simulink model "Kalman_offline_sim"  (R2022b)
settings: Solver=VariableStepAuto  StartTime=0.0  StopTime=sim_time-0.02  RelTol=1e-3
values from neighbouring files (symbols this model uses):
  A_d = (eye(size(A))+Ts*A)    [Kalman_offline.m]    (also in Main_sim.m; Startup_labview.m)
  B_d = Ts*B    [Kalman_offline.m]    (also in Main_sim.m; Startup_labview.m)
  bike_params = LoadBikeParameters(bike)    [Kalman_offline.m]    (also in Main_sim.m; Startup_labview.m)
  C1 = [1 0 0 0 0 0 0 ... (first row only)    [Kalman_offline.m]    (also in Main_sim.m; Startup_labview.m)
  C2 = [(-g+((-h_imu*g)/h)) 0 (-h_imu*(h*v^2-(g*lr*c)))*sin(lambda)/((lr+lf)*h^2)+(v^2)*sin(lambda)/(lr+lf) 0 ... (first row only)    [Kalman_offline.m]    (also in Main_sim.m; Startup_labview.m)
  D1 = [0 0 (-h_imu*lr*v)/((lr+lf)*h) 0 0 0 0]'    [Kalman_offline.m]    (also in Main_sim.m; Startup_labview.m)
  D2 = [(-h_imu*lr*v)/((lr+lf)*h) 0 0 0 0]'    [Kalman_offline.m]    (also in Main_sim.m; Startup_labview.m)
  gps_delay = 5    [Kalman_offline.m]
  initial_state_estimate = initial_state    [Kalman_offline.m]    (also in Main_sim.m)
  Kalman_gain1 = Kalman_gain1'    [Kalman_offline.m]    (also in Main_sim.m; Startup_labview.m)
  Kalman_gain2 = Kalman_gain1(4:7,3:7)    [Kalman_offline.m]    (also in Main_sim.m; Startup_labview.m)
  T = Rz*Ry*Rx    [Kalman_offline.m]    (also in Main_sim.m)
  Ts = 0.01    [Kalman_offline.m]    (also in Main_sim.m; Startup_labview.m)
  v = 2    [Kalman_offline.m]    (also in Main_sim.m; Startup_labview.m)
undefined symbols (not defined in the file or in its folder): initial_state
settings Model: Creator=gaizk  LastModifiedBy=levi1
settings SolverCC: AlgebraicLoopSolver=TrustRegion

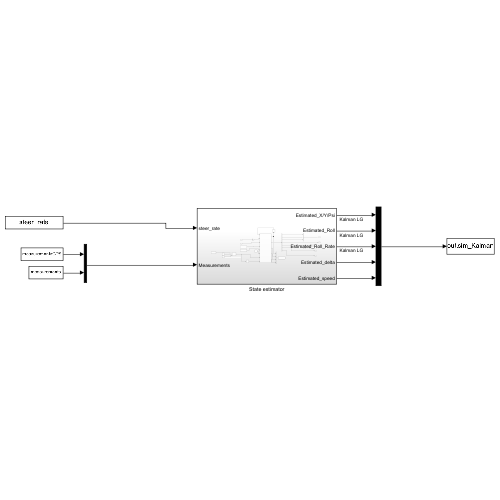
[thumbnail: Simulink's stored preview of the top-level diagram]
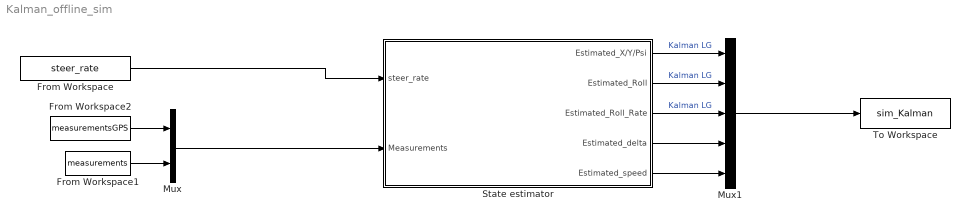
== system Kalman_offline_sim ==
  From Workspace : FromWorkspace  VariableName=steer_rate  SampleTime=Ts  OutputAfterFinalValue=Holding final value
  From Workspace1 : FromWorkspace  VariableName=measurements  SampleTime=Ts  OutputAfterFinalValue=Holding final value
  From Workspace2 : FromWorkspace  VariableName=measurementsGPS  SampleTime=Ts  OutputAfterFinalValue=Holding final value
  Mux : Mux  Inputs=2
  Mux1 : Mux  Inputs=5
  State estimator : Subsystem
  To Workspace : ToWorkspace  VariableName=sim_Kalman  SaveFormat=Timeseries  SampleTime=-1
  wires:
  From Workspace2/1 -> Mux/1
  From Workspace1/1 -> Mux/2
  State estimator/2(Estimated_Roll) -> Mux1/2  "Kalman LG"
  State estimator/1(Estimated_X/Y/Psi) -> Mux1/1  "Kalman LG"
  State estimator/3(Estimated_Roll_Rate) -> Mux1/3  "Kalman LG"
  Mux1/1 -> To Workspace/1
  State estimator/4(Estimated_delta) -> Mux1/4
  State estimator/5(Estimated_speed) -> Mux1/5
  Mux/1 -> State estimator/2(Measurements)
  From Workspace/1 -> State estimator/1(steer_rate)

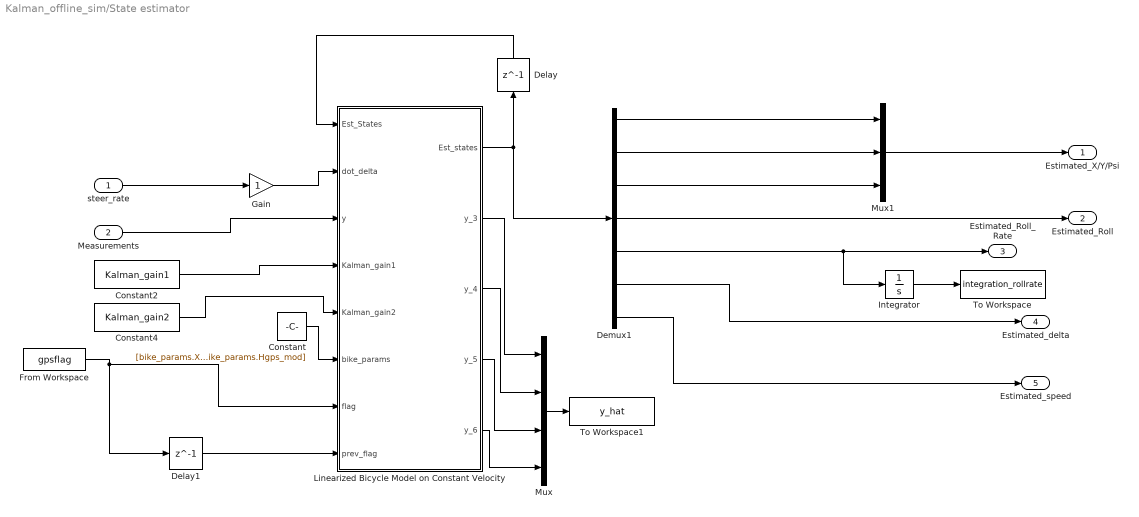
== system Kalman_offline_sim/State estimator ==
  steer_rate : Inport
  Measurements : Inport  Port=2
  Constant : Constant  Value=[bike_params.Xgps_mod bike_params.Ygps_mod bike_params.Hgps_mod]
  Constant2 : Constant  Value=Kalman_gain1  SampleTime=Ts
  Constant4 : Constant  Value=Kalman_gain2  SampleTime=Ts
  Delay : Delay  DelayLength=1  InitialCondition=[initial_state_estimate.x initial_state_estimate.y initial_state_estimate.heading initial_state.roll initial_state.roll_rate initial_state.steering v]  SampleTime=Ts
  Delay1 : Delay  DelayLength=1
  Demux1 : Demux  Outputs=7
  From Workspace : FromWorkspace  VariableName=gpsflag
  Gain : Gain
  Integrator : Integrator
  Linearized Bicycle Model on Constant Velocity : MATLAB Function  TreatAsAtomicUnit=on
  Mux : Mux
  Mux1 : Mux  Inputs=3
  To Workspace : ToWorkspace  VariableName=integration_rollrate  SaveFormat=Timeseries  SampleTime=-1
  To Workspace1 : ToWorkspace  VariableName=y_hat  SaveFormat=Timeseries  SampleTime=-1
  Estimated_X/Y/Psi : Outport  VectorParamsAs1DForOutWhenUnconnected=off
  Estimated_Roll : Outport  Port=2  VectorParamsAs1DForOutWhenUnconnected=off
  Estimated_Roll_Rate : Outport  Port=3  VectorParamsAs1DForOutWhenUnconnected=off
  Estimated_delta : Outport  Port=4  VectorParamsAs1DForOutWhenUnconnected=off
  Estimated_speed : Outport  Port=5  VectorParamsAs1DForOutWhenUnconnected=off
  wires:
  Linearized Bicycle Model on Constant Velocity/1(Est_states) -> Delay/1, Demux1/1
  Gain/1 -> Linearized Bicycle Model on Constant Velocity/2(dot_delta)
  Demux1/5 -> Integrator/1, Estimated_Roll_Rate/1
  Delay/1 -> Linearized Bicycle Model on Constant Velocity/1(Est_States)
  steer_rate/1 -> Gain/1
  Demux1/2 -> Mux1/2
  Demux1/1 -> Mux1/1
  Mux1/1 -> Estimated_X/Y/Psi/1
  Demux1/4 -> Estimated_Roll/1
  Constant2/1 -> Linearized Bicycle Model on Constant Velocity/4(Kalman_gain1)
  Constant4/1 -> Linearized Bicycle Model on Constant Velocity/5(Kalman_gain2)
  Demux1/3 -> Mux1/3
  Constant/1 -> Linearized Bicycle Model on Constant Velocity/6(bike_params)
  Measurements/1 -> Linearized Bicycle Model on Constant Velocity/3(y)
  Demux1/6 -> Estimated_delta/1
  Demux1/7 -> Estimated_speed/1
  Integrator/1 -> To Workspace/1
  Mux/1 -> To Workspace1/1
  Linearized Bicycle Model on Constant Velocity/2(y_3) -> Mux/1
  Linearized Bicycle Model on Constant Velocity/3(y_4) -> Mux/2
  Linearized Bicycle Model on Constant Velocity/4(y_5) -> Mux/3
  Linearized Bicycle Model on Constant Velocity/5(y_6) -> Mux/4
  From Workspace/1 -> Delay1/1, Linearized Bicycle Model on Constant Velocity/7(flag)
  Delay1/1 -> Linearized Bicycle Model on Constant Velocity/8(prev_flag)

== matlab function Kalman_offline_sim/State estimator/Linearized Bicycle Model on Constant Velocity ==
  data: Est_States input; dot_delta input; y input; Kalman_gain1 input; Kalman_gain2 input; bike_params input; Est_states output; flag input; prev_flag input; A_d parameter; B_d parameter; C1 parameter; C2 parameter; D1 parameter; D2 parameter; T parameter; y_3 output; y_4 output; y_5 output; y_6 output; gps_delay parameter
function [Est_states,y_3, y_4, y_5, y_6] = fcn(Est_States, dot_delta, y, Kalman_gain1, Kalman_gain2, bike_params, flag, prev_flag, A_d, B_d, C1, C2, D1, D2, T, gps_delay)
% description 
% Inputs
%   Est_States := [X Y psi phi phi_dot delta v] are global at time t 
%   dot_delta_e := effective steering rate
%   y := measurement vector
%   Kalman_gain1 := Computed state_feedback gain including GPS meas
%   Kalman_gain2 := Computed state_feedback gain excluding GPS meas
%   bike_params := vector of bike parameters + gravity
%   Ts := Estimator sampling rate
%   v := constant velocity
%   flag := [0-1] increasing counter reseted at 1. When flag == 0 means
%           that GPS measurement is available
%
% Outputs
%   Est_states : = [X Y psi phi phi_dot delta v] global at time t+1


% Transform the states to local frame 
    Est_States_l = zeros(7,1);
    
    Est_States_l(1) = Est_States(1) * cos(Est_States(3)) + Est_States(2) * sin(Est_States(3));
    Est_States_l(2) = -Est_States(1) * sin(Est_States(3)) + Est_States(2) * cos(Est_States(3));
    Est_States_l(3) = 0;        % direction of bike is aligned with X local frame
    Est_States_l(4) = Est_States(4);
    Est_States_l(5) = Est_States(5);
    Est_States_l(6) = Est_States(6);
    Est_States_l(7) = Est_States(7);

% Transform measurements to local frame
    y_l = zeros(size(y));

    y_l(1) = y(1) * cos(Est_States(3)) + y(2) * sin(Est_States(3));
    y_l(2) = -y(1) * sin(Est_States(3)) + y(2) * cos(Est_States(3)); 
    y_l(3) = y(3);
    y_l(4) = y(4);
    y_l(5) = y(5);
    y_l(6) = y(6);
    y_l(7) = y(7);
% Correct for parameter values/sensor positions
% The parameters/positions are measures by us (can differ from true values)
X_gps_mod = bike_params(1);
Y_gps_mod = bike_params(2);
H_gps_mod = bike_params(3);

y_l(1) = y_l(1) - X_gps_mod;
y_l(2) = y_l(2) - Y_gps_mod - H_gps_mod*sin(Est_States(4));

% IMU correction
raw_acc  = [0 y_l(3) 0];
raw_gyro = [y_l(4) 0 y_l(5)];

% Apply the correction to the accelerometer measurement
acc_corr = T*raw_acc';

% Apply the correction to the gyro measurement
gyro_corr = T*raw_gyro';
% Results
y_l(3) =acc_corr(2) ;
y_l(4) =gyro_corr(1) ;
y_l(5) =gyro_corr(3) ;


% Time update in local frame (from t to t+1)

    % Time update
     Est_States_l = A_d*Est_States_l + B_d*dot_delta;

    % Measurement update in local frame
     Est_states_l = zeros(7,1);

    % Sampling differentiation (Sensors rate 100Hz but GPS 10Hz)

    if flag == 0 || flag ~= prev_flag && flag > gps_delay % GPS sensors included
    
        % Select Kalman Gain
            K = Kalman_gain1;

        % Measurement prediction
            y_pred = C1*Est_States_l + D1*dot_delta;
            y_3 = y_pred(3);
            y_4 = y_pred(4);
            y_5 = y_pred(5);
            y_6 = y_pred(7);

        % Measurement update
            Est_states_l = Est_States_l + K * (y_l - y_pred);
            
    else % GPS sensors excluded
    
        % Select Kalman Gain
            K = Kalman_gain2;
    
        % Measurement prediction
            y_pred = C2*Est_States_l(4:7) + D2*dot_delta;
            y_3 = y_pred(1);
            y_4 = y_pred(2);
            y_5 = y_pred(3);
            y_6 = y_pred(5);
        % Measurement update
        Est_states_l(1) = Est_States_l(1);
        Est_states_l(2) = Est_States_l(2);
        Est_states_l(3) = Est_States_l(3);
        Est_states_l(4:7) = Est_States_l(4:7) + K * (y_l(3:7) - y_pred);
        
    end

    % Transform to global the local states at time t+1 after measurement update
    Est_states = zeros(7,1);
    Est_states(3) = Est_States(3) + Est_states_l(3);    % direction update global
    
    % Change of Coordinates from local to global frame for  states 
    Est_states(1) = Est_states_l(1) * cos(Est_States(3)) - Est_states_l(2) * sin(Est_States(3));
    Est_states(2) = Est_states_l(1) * sin(Est_States(3)) + Est_states_l(2) * cos(Est_States(3));
    Est_states(4) = Est_states_l(4);
    Est_states(5) = Est_states_l(5);
    Est_states(6) = Est_states_l(6);
    Est_states(7) = Est_states_l(7);
    
    % Heading angle between pi and -pi
    Est_states(3) = wrapToPi(Est_states(3));

end
